simulink model "SinglePipe_UT"  (R2019a)
settings: Solver=FixedStepAuto  StartTime=0.0  StopTime=200  FixedStep=0.01  RelTol=1e-3
libraries: SinglePipe_lib x24
settings Model: Creator=martin  LastModifiedBy=martin

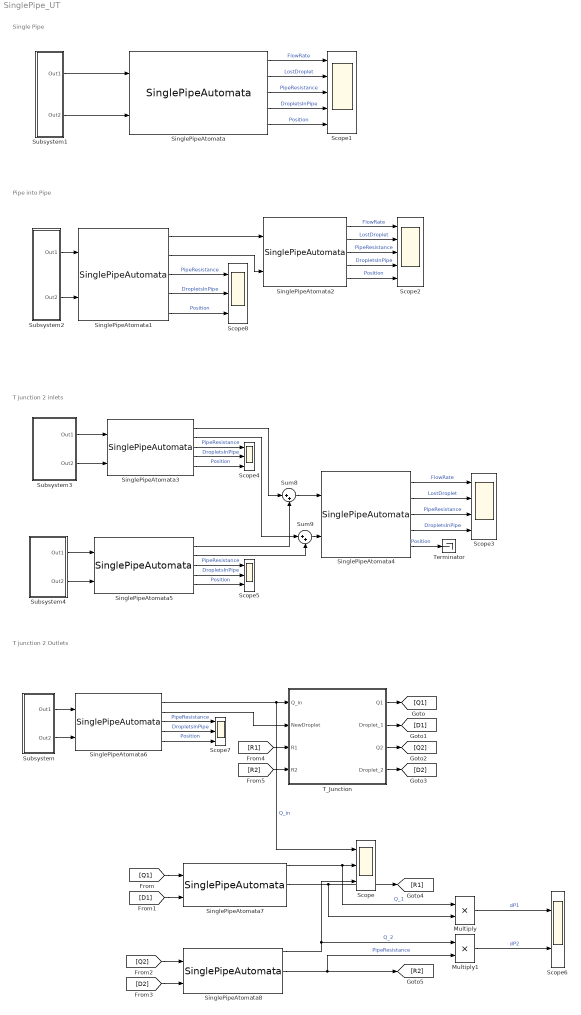
== system SinglePipe_UT ==
  note: Single Pipe
  note: Pipe into Pipe
  note: T junction 2 inlets
  note: T junction 2 Outlets
  Multiply : Product  Inputs=**
  Multiply1 : Product  Inputs=**
  Scope{,4..5,7..8} (5 alike) : Scope  NumInputPorts=3
  Scope1 : Scope  NumInputPorts=5
  Scope2 : Scope  NumInputPorts=5
  Scope3 : Scope  NumInputPorts=4
  Scope6 : Scope  NumInputPorts=2
  SinglePipeAtomata{,1,3,6} (4 alike) : SinglePipe_lib/SinglePipeAutomata  width=2  length=5  height=3  dt=0.01  R_per_droplet=1
  SinglePipeAtomata2 : SinglePipe_lib/SinglePipeAutomata  width=2  length=10  height=3  dt=0.01  R_per_droplet=1
  SinglePipeAtomata4 : SinglePipe_lib/SinglePipeAutomata  width=2  length=20  height=3  dt=0.01  R_per_droplet=1
  SinglePipeAtomata5 : SinglePipe_lib/SinglePipeAutomata  width=2  length=10  height=3  dt=0.01  R_per_droplet=1
  SinglePipeAtomata7 : SinglePipe_lib/SinglePipeAutomata  width=2  length=20  height=3  dt=0.01  R_per_droplet=1
  SinglePipeAtomata8 : SinglePipe_lib/SinglePipeAutomata  width=2  length=10  height=3  dt=0.01  R_per_droplet=1
  Subsystem : Subsystem
  Subsystem1 : Subsystem
  Subsystem2 : Subsystem
  Subsystem3 : Subsystem
  Subsystem4 : Subsystem
  Sum8 : Sum  Inputs=|++
  Sum9 : Sum  Inputs=|++
  T_Junction : Subsystem
  Terminator : Terminator
  wires:
  SinglePipeAtomata1/2 -> SinglePipeAtomata2/2
  SinglePipeAtomata1/1 -> SinglePipeAtomata2/1
  SinglePipeAtomata1/3 -> Scope8/1  "PipeResistance"
  SinglePipeAtomata/1 -> Scope1/1  "FlowRate"
  SinglePipeAtomata/2 -> Scope1/2  "LostDroplet"
  SinglePipeAtomata/3 -> Scope1/3  "PipeResistance"
  SinglePipeAtomata/4 -> Scope1/4  "DropletsInPipe"
  SinglePipeAtomata/5 -> Scope1/5  "Position"
  SinglePipeAtomata2/1 -> Scope2/1  "FlowRate"
  SinglePipeAtomata2/2 -> Scope2/2  "LostDroplet"
  SinglePipeAtomata2/5 -> Scope2/5  "Position"
  SinglePipeAtomata2/3 -> Scope2/3  "PipeResistance"
  SinglePipeAtomata2/4 -> Scope2/4  "DropletsInPipe"
  SinglePipeAtomata1/4 -> Scope8/2  "DropletsInPipe"
  SinglePipeAtomata1/5 -> Scope8/3  "Position"
  SinglePipeAtomata4/2 -> Scope3/2  "LostDroplet"
  SinglePipeAtomata4/1 -> Scope3/1  "FlowRate"
  SinglePipeAtomata4/3 -> Scope3/3  "PipeResistance"
  SinglePipeAtomata4/4 -> Scope3/4  "DropletsInPipe"
  SinglePipeAtomata3/5 -> Scope4/3  "Position"
  SinglePipeAtomata3/4 -> Scope4/2  "DropletsInPipe"
  SinglePipeAtomata3/3 -> Scope4/1  "PipeResistance"
  SinglePipeAtomata5/3 -> Scope5/1  "PipeResistance"
  SinglePipeAtomata5/4 -> Scope5/2  "DropletsInPipe"
  SinglePipeAtomata5/5 -> Scope5/3  "Position"
  Sum8/1 -> SinglePipeAtomata4/1
  SinglePipeAtomata3/1 -> Sum8/1
  SinglePipeAtomata5/1 -> Sum8/2
  Sum9/1 -> SinglePipeAtomata4/2
  SinglePipeAtomata5/2 -> Sum9/2
  SinglePipeAtomata3/2 -> Sum9/1
  SinglePipeAtomata4/5 -> Terminator/1  "Position"
  SinglePipeAtomata6/4 -> Scope7/2  "DropletsInPipe"
  SinglePipeAtomata6/5 -> Scope7/3  "Position"
  SinglePipeAtomata6/3 -> Scope7/1  "PipeResistance"
  Subsystem/1(Out1) -> SinglePipeAtomata6/1
  Subsystem/2(Out2) -> SinglePipeAtomata6/2
  Subsystem1/1(Out1) -> SinglePipeAtomata/1
  Subsystem1/2(Out2) -> SinglePipeAtomata/2
  Subsystem2/1(Out1) -> SinglePipeAtomata1/1
  Subsystem2/2(Out2) -> SinglePipeAtomata1/2
  Subsystem3/1(Out1) -> SinglePipeAtomata3/1
  Subsystem3/2(Out2) -> SinglePipeAtomata3/2
  Subsystem4/1(Out1) -> SinglePipeAtomata5/1
  Subsystem4/2(Out2) -> SinglePipeAtomata5/2
  SinglePipeAtomata6/1 -> Scope/1, T_Junction/1(Q_in)  "Q_in"
  SinglePipeAtomata6/2 -> T_Junction/2(NewDroplet)
  T_Junction/1(Q1) -> [Q1]
  T_Junction/2(Droplet_1) -> [D1]
  SinglePipeAtomata7/3 -> Multiply/2, [R1]
  SinglePipeAtomata8/3 -> Multiply1/2, [R2]  "PipeResistance"
  T_Junction/3(Q2) -> [Q2]
  T_Junction/4(Droplet_2) -> [D2]
  [R1] -> T_Junction/3(R1)
  [R2] -> T_Junction/4(R2)
  [D2] -> SinglePipeAtomata8/2
  [Q2] -> SinglePipeAtomata8/1
  [D1] -> SinglePipeAtomata7/2
  [Q1] -> SinglePipeAtomata7/1
  SinglePipeAtomata7/1 -> Multiply/1, Scope/2  "Q_1"
  SinglePipeAtomata8/1 -> Multiply1/1, Scope/3  "Q_2"
  Multiply/1 -> Scope6/1  "dP1"
  Multiply1/1 -> Scope6/2  "dP2"

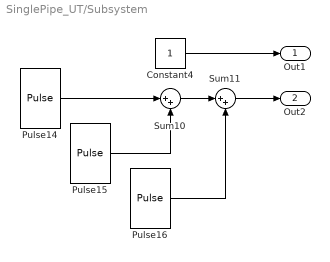
== system SinglePipe_UT/Subsystem ==
  Constant4 : Constant
  Pulse14 : SinglePipe_lib/Pulse  time=1  duration=0.01
  Pulse15 : SinglePipe_lib/Pulse  time=15  duration=0.01
  Pulse16 : SinglePipe_lib/Pulse  time=20  duration=0.01
  Sum10 : Sum  Inputs=|++
  Sum11 : Sum  Inputs=|++
  Out1 : Outport
  Out2 : Outport  Port=2
  wires:
  Sum11/1 -> Out2/1
  Pulse15/1 -> Sum10/2
  Constant4/1 -> Out1/1
  Pulse14/1 -> Sum10/1
  Pulse16/1 -> Sum11/2
  Sum10/1 -> Sum11/1

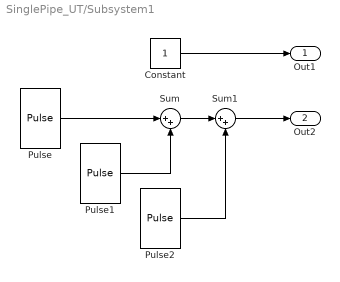
== system SinglePipe_UT/Subsystem1 ==
  Constant : Constant
  Pulse : SinglePipe_lib/Pulse  time=1  duration=0.01
  Pulse1 : SinglePipe_lib/Pulse  time=15  duration=0.01
  Pulse2 : SinglePipe_lib/Pulse  time=1.5  duration=0.01
  Sum : Sum  Inputs=|++
  Sum1 : Sum  Inputs=|++
  Out1 : Outport
  Out2 : Outport  Port=2
  wires:
  Pulse1/1 -> Sum/2
  Pulse2/1 -> Sum1/2
  Pulse/1 -> Sum/1
  Sum1/1 -> Out2/1
  Constant/1 -> Out1/1
  Sum/1 -> Sum1/1

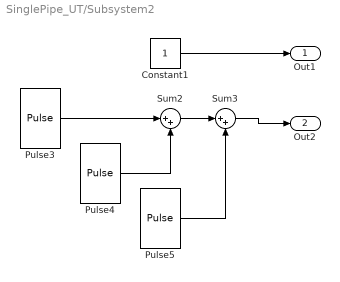
== system SinglePipe_UT/Subsystem2 ==
  Constant1 : Constant
  Pulse3 : SinglePipe_lib/Pulse  time=1  duration=0.01
  Pulse4 : SinglePipe_lib/Pulse  time=15  duration=0.01
  Pulse5 : SinglePipe_lib/Pulse  time=20  duration=0.01
  Sum2 : Sum  Inputs=|++
  Sum3 : Sum  Inputs=|++
  Out1 : Outport
  Out2 : Outport  Port=2
  wires:
  Sum3/1 -> Out2/1
  Pulse4/1 -> Sum2/2
  Pulse3/1 -> Sum2/1
  Sum2/1 -> Sum3/1
  Pulse5/1 -> Sum3/2
  Constant1/1 -> Out1/1

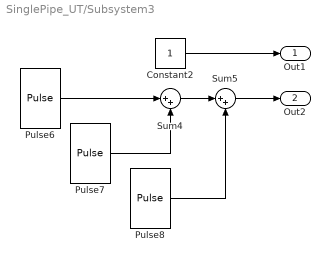
== system SinglePipe_UT/Subsystem3 ==
  Constant2 : Constant
  Pulse6 : SinglePipe_lib/Pulse  time=1  duration=0.01
  Pulse7 : SinglePipe_lib/Pulse  time=15  duration=0.01
  Pulse8 : SinglePipe_lib/Pulse  time=20  duration=0.01
  Sum4 : Sum  Inputs=|++
  Sum5 : Sum  Inputs=|++
  Out1 : Outport
  Out2 : Outport  Port=2
  wires:
  Pulse8/1 -> Sum5/2
  Pulse7/1 -> Sum4/2
  Sum4/1 -> Sum5/1
  Pulse6/1 -> Sum4/1
  Sum5/1 -> Out2/1
  Constant2/1 -> Out1/1

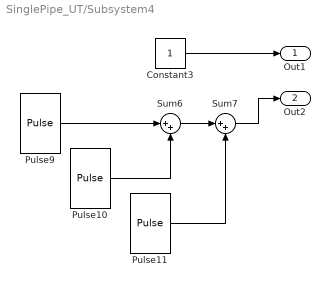
== system SinglePipe_UT/Subsystem4 ==
  Constant3 : Constant
  Pulse10 : SinglePipe_lib/Pulse  time=15  duration=0.01
  Pulse11 : SinglePipe_lib/Pulse  time=20  duration=0.01
  Pulse9 : SinglePipe_lib/Pulse  time=1  duration=0.01
  Sum6 : Sum  Inputs=|++
  Sum7 : Sum  Inputs=|++
  Out1 : Outport
  Out2 : Outport  Port=2
  wires:
  Sum6/1 -> Sum7/1
  Pulse10/1 -> Sum6/2
  Pulse11/1 -> Sum7/2
  Constant3/1 -> Out1/1
  Pulse9/1 -> Sum6/1
  Sum7/1 -> Out2/1

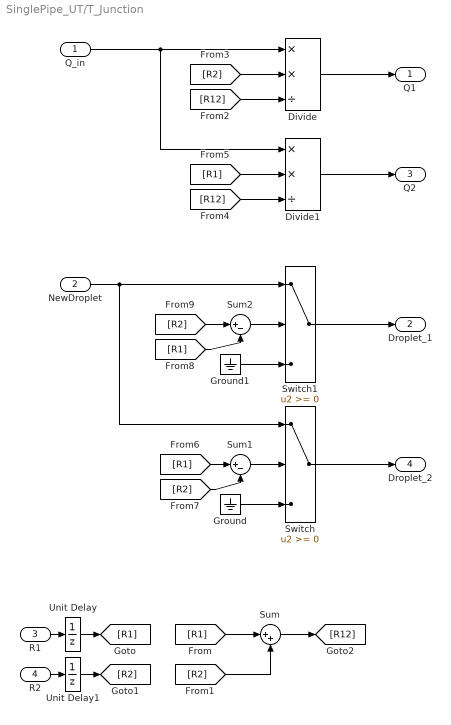
== system SinglePipe_UT/T_Junction ==
  Q_in : Inport
  NewDroplet : Inport  Port=2
  R1 : Inport  Port=3
  R2 : Inport  Port=4
  Divide : Product  Inputs=**/
  Divide1 : Product  Inputs=**/
  Ground : Ground
  Ground1 : Ground
  Sum : Sum  Inputs=|++
  Sum1 : Sum  Inputs=|+-
  Sum2 : Sum  Inputs=|+-
  Switch : Switch
  Switch1 : Switch
  Unit Delay : UnitDelay  SampleTime=-1  HasFrameUpgradeWarning=on
  Unit Delay1 : UnitDelay  SampleTime=-1  HasFrameUpgradeWarning=on
  Q1 : Outport
  Droplet_1 : Outport  Port=2
  Q2 : Outport  Port=3
  Droplet_2 : Outport  Port=4
  wires:
  R1/1 -> Unit Delay/1
  R2/1 -> Unit Delay1/1
  [R1] -> Sum/1
  [R2] -> Sum/2
  Sum/1 -> [R12]
  Unit Delay/1 -> [R1]
  Unit Delay1/1 -> [R2]
  [R12] -> Divide/3
  [R2] -> Divide/2
  Q_in/1 -> Divide1/1, Divide/1
  [R1] -> Divide1/2
  [R12] -> Divide1/3
  Divide1/1 -> Q2/1
  Divide/1 -> Q1/1
  Ground/1 -> Switch/3
  Switch/1 -> Droplet_2/1
  [R1] -> Sum1/1
  [R2] -> Sum1/2
  Sum1/1 -> Switch/2
  Ground1/1 -> Switch1/3
  NewDroplet/1 -> Switch1/1, Switch/1
  Switch1/1 -> Droplet_1/1
  Sum2/1 -> Switch1/2
  [R2] -> Sum2/1
  [R1] -> Sum2/2
